simulink model "task3"  (R2023b)
settings: Solver=FixedStepDiscrete  StartTime=0.0  StopTime=10  FixedStep=5e-5  RelTol=1e-3
PreLoadFcn:
  | Simulink.defineIntEnumType('windowCommand', {'Off','Speed1','Speed2','Speed3'},[0,1,2,3])
undefined symbols (not defined in the file): windowCommand
libraries: simulink x5, slpidlib x1
settings Model: Creator=kz1nz0  LastModifiedBy=aleks

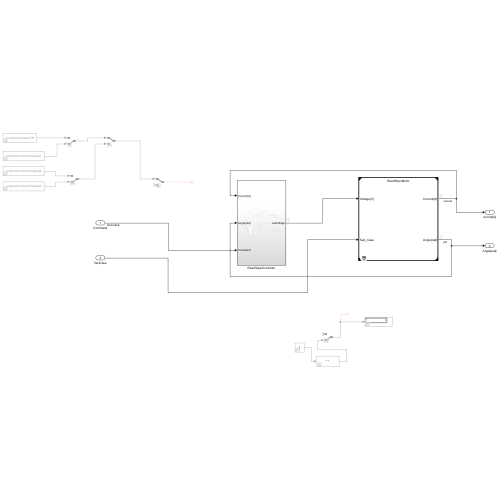
[thumbnail: Simulink's stored preview of the top-level diagram]
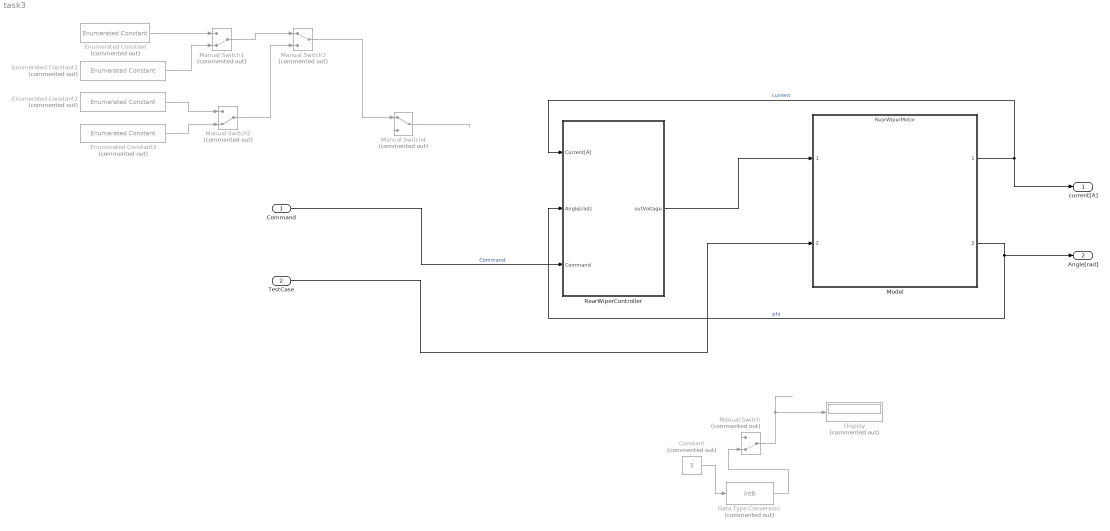
== system task3 ==
  Command : Inport  OutDataTypeStr=Enum: windowCommand
  TestCase : Inport  Port=2  OutDataTypeStr=int8
  Constant : Constant  Commented=on  Value=3
  Data Type Conversion : DataTypeConversion  Commented=on  OutDataTypeStr=int8  SaturateOnIntegerOverflow=off  RndMeth=Floor
  Display : Display  Commented=on
  Enumerated Constant : simulink/Sources/Enumerated Constant  Commented=on  OutDataTypeStr=Enum: windowCommand  Value=windowCommand.Off  SampleTime=inf
  Enumerated Constant1 : simulink/Sources/Enumerated Constant  Commented=on  OutDataTypeStr=Enum: windowCommand  Value=windowCommand.Speed1  SampleTime=inf
  Enumerated Constant2 : simulink/Sources/Enumerated Constant  Commented=on  OutDataTypeStr=Enum: windowCommand  Value=windowCommand.Speed2  SampleTime=inf
  Enumerated Constant3 : simulink/Sources/Enumerated Constant  Commented=on  OutDataTypeStr=Enum: windowCommand  Value=windowCommand.Speed3  SampleTime=inf
  Manual Switch : ManualSwitch  Commented=on  CurrentSetting=0
  Manual Switch1 : ManualSwitch  Commented=on  CurrentSetting=0
  Manual Switch2 : ManualSwitch  Commented=on  CurrentSetting=0
  Manual Switch3 : ManualSwitch  Commented=on
  Manual Switch4 : ManualSwitch  Commented=on
  Model : ModelReference  ModelNameDialog=RearWiperMotor.slxp  ModelReferenceVersion=19.15  CopyOfModelProtected=on
  RearWiperController : Subsystem
  current[A] : Outport
  Angle[rad] : Outport  Port=2
  wires:
  Command/1 -> RearWiperController/3(Command)  "Command"
  TestCase/1 -> Model/2
  Model/1 -> current[A]/1, RearWiperController/1(Current[A])  "current"
  Model/2 -> RearWiperController/2(Angle[rad]), Angle[rad]/1  "phi"
  RearWiperController/1(outVoltage) -> Model/1
  Constant/1 -> Data Type Conversion/1
  Data Type Conversion/1 -> Manual Switch/2
  Manual Switch/1 -> Display/1
  Enumerated Constant/1 -> Manual Switch1/1
  Manual Switch1/1 -> Manual Switch3/1
  Enumerated Constant3/1 -> Manual Switch2/2
  Manual Switch2/1 -> Manual Switch3/2
  Enumerated Constant1/1 -> Manual Switch1/2
  Enumerated Constant2/1 -> Manual Switch2/1
  Manual Switch3/1 -> Manual Switch4/1
  Manual Switch4/1 -> ?

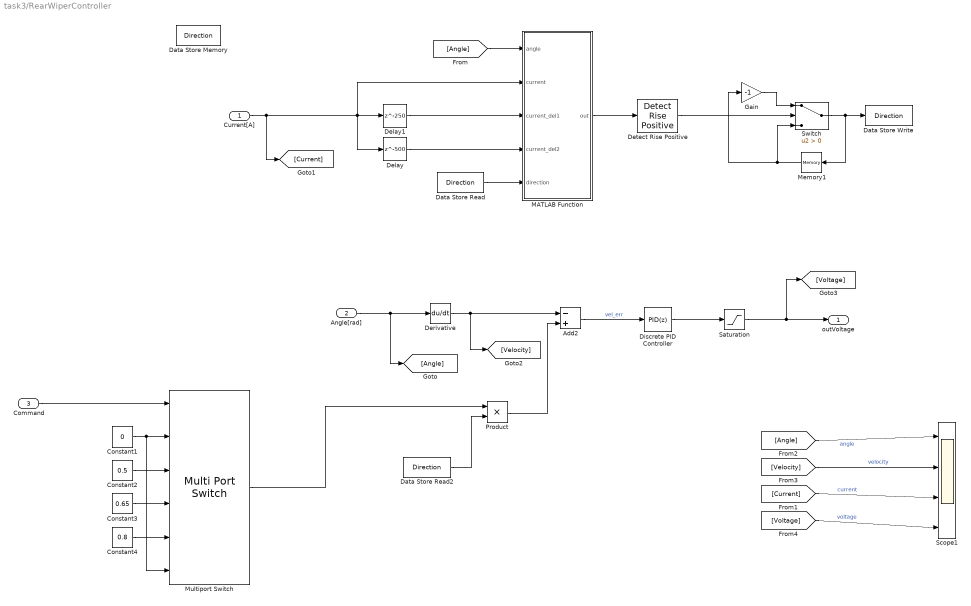
== system task3/RearWiperController ==
  Current[A] : Inport
  Angle[rad] : Inport  Port=2
  Command : Inport  Port=3  OutDataTypeStr=Enum: windowCommand
  Add2 : Sum  Inputs=-+
  Constant1 : Constant  Value=0
  Constant2 : Constant  Value=0.5
  Constant3 : Constant  Value=0.65
  Constant4 : Constant  Value=0.8
  Data Store Memory : DataStoreMemory  DataStoreName=Direction  WriteAfterWriteMsg=warning  InitialValue=1  ShowAdditionalParam=off
  Data Store Read : DataStoreRead  DataStoreName=Direction  IndexOptions=Index vector (dialog)  Indices=1  OutputSizes=1
  Data Store Read2 : DataStoreRead  DataStoreName=Direction  IndexOptions=Index vector (dialog)  Indices=1  OutputSizes=1
  Data Store Write : DataStoreWrite  DataStoreName=Direction  IndexOptions=Index vector (dialog)  Indices=1  OutputSizes=1
  Delay : Delay  DelayLength=500
  Delay1 : Delay  DelayLength=250
  Derivative : Derivative
  Detect Rise Positive : simulink/Logic and Bit Operations/Detect Rise Positive  vinit=0  OutDataTypeStr=boolean
  Discrete PID Controller : slpidlib/PID Controller  Controller=PID  Form=Parallel  TimeDomain=Discrete-time  UseExternalTs=off  SampleTime=-1  IntegratorMethod=Forward Euler  FilterMethod=Forward Euler  ControllerParametersSource=internal  P=70  I=40  UseKiTs=off  D=5  N=100  UseFilter=on  TunerSelectOption=Frequency Response Based  InitialConditionSource=internal  InitialConditionForIntegrator=0  InitialConditionForFilter=0  DifferentiatorICPrevScaledInput=0  ExternalReset=none  TrackingMode=off  Kt=1  LimitOutput=off  SatLimitsSource=internal  UpperSaturationLimit=inf  LowerSaturationLimit=-inf  LinearizeAsGain=off  AntiWindupMode=none  Kb=1  LimitIntegrator=off  UpperIntegratorSaturationLimit=inf  LowerIntegratorSaturationLimit=-inf  POutMin=[]  POutMax=[]  IOutMin=[]  IOutMax=[]  DOutMin=[]  DOutMax=[]  NOutMin=[]  NOutMax=[]  SumOutMin=[]  SumOutMax=[]  SaturationOutMin=[]  SaturationOutMax=[]  PParamMin=[]  PParamMax=[]  IParamMin=[]  IParamMax=[]  DParamMin=[]  DParamMax=[]  NParamMin=[]  NParamMax=[]  KbParamMin=[]  KbParamMax=[]  KtParamMin=[]  KtParamMax=[]  KbOutMin=[]  KbOutMax=[]  KtOutMin=[]  KtOutMax=[]  IntegratorOutMin=[]  IntegratorOutMax=[]  FilterOutMin=[]  FilterOutMax=[]  SumI1OutMin=[]  SumI1OutMax=[]  SumI2OutMin=[]  SumI2OutMax=[]  SumI3OutMin=[]  SumI3OutMax=[]  SumI4OutMin=[]  SumI4OutMax=[]  SumDOutMin=[]  SumDOutMax=[]  DifferentiatorOutMin=[]  DifferentiatorOutMax=[]  FilterDiffOutCoefMin=[]  FilterDiffOutCoefMax=[]  ReciprocalOutMin=[]  ReciprocalOutMax=[]  SumDenOutMin=[]  SumDenOutMax=[]  SumNumOutMin=[]  SumNumOutMax=[]  DivideOutMin=[]  DivideOutMax=[]  UdiffTsProdOutMin=[]  UdiffTsProdOutMax=[]  NTsProdOutMin=[]  NTsProdOutMax=[]  UintegralTsProdOutMin=[]  UintegralTsProdOutMax=[]  UngainTsProdOutMin=[]  UngainTsProdOutMax=[]  ClampingZeroOutDataTypeStr=Inherit: Inherit via back propagation  ClampingZeroOutMin=[]  ClampingZeroOutMax=[]  FilterDenConstantOutDataTypeStr=Inherit: Inherit via back propagation  FilterDenConstantOutMin=[]  FilterDenConstantOutMax=[]  PCopyOutDataTypeStr=Inherit: Inherit via back propagation  PCopyOutMin=[]  PCopyOutMax=[]  NCopyOutDataTypeStr=Inherit: Inherit via back propagation  NCopyOutMin=[]  NCopyOutMax=[]  IntegratorContinuousStateAttributes=''  IntegratorStateMustResolveToSignalObject=off  IntegratorRTWStateStorageClass=Auto  FilterContinuousStateAttributes=''  FilterStateMustResolveToSignalObject=off  FilterRTWStateStorageClass=Auto  ParallelPVariant=InternalParameters  IdealPVariant=Disabled  IVariant=InternalParameters  DVariant=InternalParameters  IntegratorVariant=Discrete  SatVariant=Disabled  AWVariant=Passthrough  PCopyVariant=Disabled  TRVariant=Disabled  FdbkBlocksVariant=Forward  IdealPFdbkVariant=Disabled  SatFdbkVariant=Disabled  DerivativeFilterVariant=ForwardEulerFilter  NVariant=InternalParameters  NCopyVariant=Disabled  FilterICVariant=InternalICsFilter  IntegratorICVariant=InternalICs  ExternalResetVariant=Disabled  TRSumVariant=Passthrough  SumFdbkVariant=Disabled  SumVariant=Sum_PID  TsampFilterVariant=InternalTs  TsampNgainVariant=Passthrough  TsampIntegralVariant=Disabled_SignalSpec  ExternalSaturationOutDataTypeStr=Inherit: Same as second input
      settings: LibrarySourceBlock=simulink/Discrete/Discrete PID Controller
  Gain : Gain  Gain=-1
  MATLAB Function : MATLAB Function  TreatAsAtomicUnit=on
  Memory1 : Memory  InitialCondition=1
  Multiport Switch : MultiPortSwitch  DataPortOrder=Specify indices  DataPortIndices={windowCommand.Off, windowCommand.Speed1, windowCommand.Speed2, windowCommand.Speed3}  DataPortForDefault=Additional data port  SaturateOnIntegerOverflow=off  InputSameDT=off
  Product : Product
  Saturation : Saturate  UpperLimit=12  LowerLimit=-12
  Scope1 : Scope  NumInputPorts=4
  Switch : Switch  Criteria=u2 > Threshold  SaturateOnIntegerOverflow=off  InputSameDT=off
  outVoltage : Outport
  wires:
  Angle[rad]/1 -> Derivative/1, [Angle]
  Multiport Switch/1 -> Product/1
  Constant2/1 -> Multiport Switch/3
  Constant3/1 -> Multiport Switch/4
  Constant4/1 -> Multiport Switch/5
  Constant1/1 -> Multiport Switch/6, Multiport Switch/2
  Saturation/1 -> outVoltage/1, [Voltage]
  Derivative/1 -> [Velocity], Add2/1
  Command/1 -> Multiport Switch/1
  Detect Rise Positive/1 -> Switch/2
  Switch/1 -> Memory1/1, Data Store Write/1
  Memory1/1 -> Gain/1, Switch/3
  Gain/1 -> Switch/1
  Delay1/1 -> MATLAB Function/3(current_del1)
  Delay/1 -> MATLAB Function/4(current_del2)
  [Angle] -> MATLAB Function/1(angle)
  Data Store Read/1 -> MATLAB Function/5(direction)
  MATLAB Function/1(out) -> Detect Rise Positive/1
  Product/1 -> Add2/2
  Data Store Read2/1 -> Product/2
  Add2/1 -> Discrete PID Controller/1  "vel_err"
  Discrete PID Controller/1 -> Saturation/1
  [Angle] -> Scope1/1  "angle"
  [Velocity] -> Scope1/2  "velocity"
  [Voltage] -> Scope1/4  "voltage"
  [Current] -> Scope1/3  "current"
  Current[A]/1 -> Delay/1, MATLAB Function/2(current), Delay1/1, [Current]

== matlab function task3/RearWiperController/MATLAB Function ==
  data: angle input; current input; out output; current_del1 input; current_del2 input; direction input
function out = change_direction(angle, current, current_del1, current_del2, direction)

% Funkcja wykrywa moment zwiększenia obciążenia i zmienia wartość zmiennej
% przechowującej informacje o kierunku obrotu

curr_diff_tresh = 0.5;  % [A]
angle_tresh_pos = 2;    % [rad]
angle_tresh_neg = 1;    % [rad]

% direction = -1  -> obrót w lewo (ujemne napięcie)
% direction = 1  -> obrót w prawo (dodatnie napięcie)

if(direction == -1)
    out = (abs(current - current_del1) >= abs(current_del1 - current_del2) && abs(current - current_del1) > curr_diff_tresh) && angle < angle_tresh_neg;

elseif(direction == 1)
    out = (abs(current - current_del1) >= abs(current_del1 - current_del2) && abs(current - current_del1) > curr_diff_tresh) && angle > angle_tresh_pos;

else
    out = true;

end
